simulink model "rtwdemo_examplemain"  (Simulink 7.6)
settings: Solver=FixedStepDiscrete  SolverMode=MultiTasking  StartTime=0.0  StopTime=10.0  FixedStep=1  RelTol=1e-3
undefined symbols (not defined in the file or in its folder): DiscIntNeverNeededParam
libraries: rtwdemowidgets x2
Description:
  | Customizing a Main Program for Your Target
settings Model: Creator=The MathWorks Inc.  ExtModeArmWhenConnect=off  ExtModeAutoUpdateStatusClock=off
settings MATStruct: SampleTime=1  Offset=0  Priority=[20.0]
settings DataIOCC: SaveOutput=off  SaveTime=off  SignalLoggingName=sigsOut
settings OptimizationCC: InlineParams=on  InlineInvariantSignals=on  PassReuseOutputArgsAs=Individual arguments  StateBitsets=on  DataBitsets=on  UseTempVars=on  ZeroExternalMemoryAtStartup=off  ZeroInternalMemoryAtStartup=off  NoFixptDivByZeroProtection=on  EfficientFloat2IntCast=on  EfficientMapNaN2IntZero=off  OptimizeModelRefInitCode=on  LifeSpan=1
settings DebuggingCC: CheckExecutionContextPreStartOutputMsg=on  CheckExecutionContextRuntimeOutputMsg=on  SolverPrmCheckMsg=none  UnconnectedInputMsg=none  UnconnectedOutputMsg=none  UnconnectedLineMsg=none  StrictBusMsg=ErrorOnBusTreatedAsVector
settings HardwareCC: ProdIntDivRoundTo=Zero  ProdEndianess=LittleEndian  ProdHWDeviceType=Generic->32-bit Embedded Processor  TargetHWDeviceType=Generic->32-bit Embedded Processor
settings RTWCC: SystemTargetFile=ert.tlc  TLCOptions=-p0 -aWarnNonSaturatedBlocks=0  TemplateMakefile=ert_default_tmf  GenerateReport=on  RTWVerbose=off  ProcessScript=ert_make_rtw_hook  IncludeHyperlinkInReport=on  LaunchReport=on
settings CodeAppCC: ForceParamTrailComments=on  IgnoreCustomStorageClasses=off  IgnoreTestpoints=on  SimulinkDataObjDesc=on  CustomSymbolStrGlobalVar=rt$N$M  CustomSymbolStrType=$N$M  CustomSymbolStrFcn=$N$M$F  CustomSymbolStrMacro=$N$M  InsertBlockDesc=on
settings ERTTargetCC: TargetFcnLib=ansi_tfl_tmw.mat  MultiwordLength=2048  GenerateSampleERTMain=on  IncludeMdlTerminateFcn=off  SupportNonFinite=off  InlinedParameterPlacement=NonHierarchical  ERTCustomFileTemplate=example_file_process.tlc  ConvertIfToSwitch=off

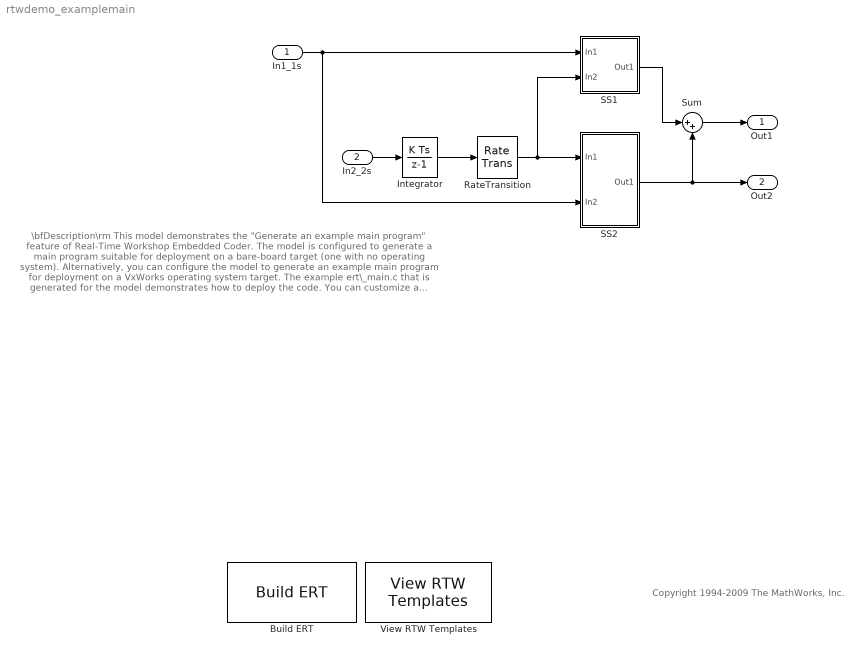
== system rtwdemo_examplemain ==
  note: \bfDescription\rm
      | This model demonstrates the "Generate an example main program" feature of Real-Time Workshop
      | Embedded Coder.  The model is configured to generate a main program suitable for deployment
      | on a bare-board target (one with no operating system).  Alternatively, you can configure the
      | model to generate an example main program for deployment on a VxWorks operating system target.
      | The example ert\_main.c that is generated for the model demonstrates how to deploy the code.
      |
      | You can customize a generated main program using the Real-Time Workshop Embedded Coder
      | "File customization template," which is located on the Real-Time Workshop Templates page.
      | See the Real-Time Workshop Embedded Coder documentation for a description of this feature.
      |
      | \bfInstructions\rm
      | To select the "Generate an example main program" option,
      | 1. From the menu bar, choose Simulation > Configuration Parameters.
      | 2. Select the Real-Time Workshop Templates page.
      | 3. Select "Generate an example main program."
      | 4. Configure "Target operating system."
  note: Copyright 1994-2009 The MathWorks, Inc.
  In1_1s : Inport  OutDataTypeStr=double  PortDimensions=1  SampleTime=1
  In2_2s : Inport  Port=2  OutDataTypeStr=double  PortDimensions=1  SampleTime=2
  Build ERT : rtwdemowidgets/Build ERT  SystemSampleTime=-1  attrib_overrides={'TargetOS'}
  Integrator : DiscreteIntegrator  InitialConditionMode=State only (most efficient)  SampleTime=-1  SaturateOnIntegerOverflow=on  ICPrevOutput=DiscIntNeverNeededParam  ICPrevScaledInput=DiscIntNeverNeededParam
  RateTransition : RateTransition
  SS1 : Subsystem  TreatAsAtomicUnit=on
  SS2 : Subsystem  TreatAsAtomicUnit=on
  Sum : Sum  Inputs=|++  SaturateOnIntegerOverflow=on  InputSameDT=on  OutDataTypeStr=Inherit: Same as first input
  View RTW Templates : rtwdemowidgets/View RTW Templates  SystemSampleTime=-1
  Out1 : Outport
  Out2 : Outport  Port=2
  wires:
  In1_1s/1 -> SS1/1(In1), SS2/2(In2)
  In2_2s/1 -> Integrator/1
  SS2/1(Out1) -> Out2/1, Sum/2
  SS1/1(Out1) -> Sum/1
  Sum/1 -> Out1/1
  RateTransition/1 -> SS2/1(In1), SS1/2(In2)
  Integrator/1 -> RateTransition/1

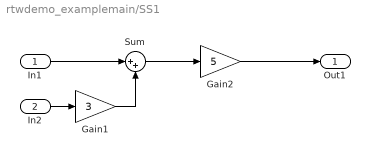
== system rtwdemo_examplemain/SS1 ==
  In1 : Inport
  In2 : Inport  Port=2
  Gain1 : Gain  Gain=3  SaturateOnIntegerOverflow=on  OutDataTypeStr=Inherit: Same as input  ParamDataTypeStr=Inherit: Same as input
  Gain2 : Gain  Gain=5  SaturateOnIntegerOverflow=on  OutDataTypeStr=Inherit: Same as input  ParamDataTypeStr=Inherit: Same as input
  Sum : Sum  Inputs=|++  SaturateOnIntegerOverflow=on  InputSameDT=on  OutDataTypeStr=Inherit: Same as first input
  Out1 : Outport
  wires:
  In1/1 -> Sum/1
  Sum/1 -> Gain2/1
  In2/1 -> Gain1/1
  Gain2/1 -> Out1/1
  Gain1/1 -> Sum/2

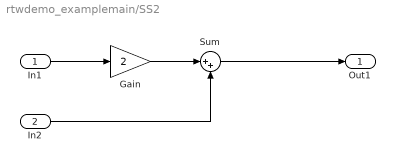
== system rtwdemo_examplemain/SS2 ==
  In1 : Inport
  In2 : Inport  Port=2
  Gain : Gain  Gain=2  SaturateOnIntegerOverflow=on  OutDataTypeStr=Inherit: Same as input  ParamDataTypeStr=Inherit: Same as input
  Sum : Sum  Inputs=|++  SaturateOnIntegerOverflow=on  InputSameDT=on  OutDataTypeStr=Inherit: Same as first input
  Out1 : Outport
  wires:
  In1/1 -> Gain/1
  Gain/1 -> Sum/1
  Sum/1 -> Out1/1
  In2/1 -> Sum/2
